simulink model "Grid_Forming_Converters_Microgrid_Github"  (R2020b)
settings: Solver=VariableStepAuto  StartTime=0.0  StopTime=1  RelTol=1e-3
values from neighbouring files (symbols this model uses):
  C_fi_1DG = 50*10^-6    (= 5e-05)    [Script_Primary_Secondary_Controller_GITHUB.m]
  C_fi_2DG = 50*10^-6    (= 5e-05)    [Script_Primary_Secondary_Controller_GITHUB.m]
  C_fi_3DG = 50*10^-6    (= 5e-05)    [Script_Primary_Secondary_Controller_GITHUB.m]
  C_fi_4DG = 50*10^-6    (= 5e-05)    [Script_Primary_Secondary_Controller_GITHUB.m]
  Kff_i_1DG = 0.75    [Script_Primary_Secondary_Controller_GITHUB.m]
  Kff_i_2DG = 0.75    [Script_Primary_Secondary_Controller_GITHUB.m]
  Kff_i_3DG = 0.75    [Script_Primary_Secondary_Controller_GITHUB.m]
  Kff_i_4DG = 0.75    [Script_Primary_Secondary_Controller_GITHUB.m]
  ki = 142500    [Script_Primary_Secondary_Controller_GITHUB.m]
  Kii_1DG = 20000    [Script_Primary_Secondary_Controller_GITHUB.m]
  Kii_2DG = 20000    [Script_Primary_Secondary_Controller_GITHUB.m]
  Kii_3DG = 16000    [Script_Primary_Secondary_Controller_GITHUB.m]
  Kii_4DG = 16000    [Script_Primary_Secondary_Controller_GITHUB.m]
  Kiv_1DG = 420    [Script_Primary_Secondary_Controller_GITHUB.m]
  Kiv_2DG = 420    [Script_Primary_Secondary_Controller_GITHUB.m]
  Kiv_3DG = 390    [Script_Primary_Secondary_Controller_GITHUB.m]
  Kiv_4DG = 390    [Script_Primary_Secondary_Controller_GITHUB.m]
  kp = 285    [Script_Primary_Secondary_Controller_GITHUB.m]
  Kpi_1DG = 15    [Script_Primary_Secondary_Controller_GITHUB.m]
  Kpi_2DG = 15    [Script_Primary_Secondary_Controller_GITHUB.m]
  Kpi_3DG = 10.5    [Script_Primary_Secondary_Controller_GITHUB.m]
  Kpi_4DG = 10.5    [Script_Primary_Secondary_Controller_GITHUB.m]
  Kpv_1DG = 0.1    [Script_Primary_Secondary_Controller_GITHUB.m]
  Kpv_2DG = 0.1    [Script_Primary_Secondary_Controller_GITHUB.m]
  Kpv_3DG = 0.05    [Script_Primary_Secondary_Controller_GITHUB.m]
  Kpv_4DG = 0.05    [Script_Primary_Secondary_Controller_GITHUB.m]
  L_ci_1DG = 0.35*10^-3    (= 0.00035)    [Script_Primary_Secondary_Controller_GITHUB.m]
  L_ci_2DG = 0.35*10^-3    (= 0.00035)    [Script_Primary_Secondary_Controller_GITHUB.m]
  L_fi_1DG = 1.35*10^-3    (= 0.00135)    [Script_Primary_Secondary_Controller_GITHUB.m]
  L_fi_2DG = 1.35*10^-3    (= 0.00135)    [Script_Primary_Secondary_Controller_GITHUB.m]
  L_fi_3DG = 1.35*10^-3    (= 0.00135)    [Script_Primary_Secondary_Controller_GITHUB.m]
  L_fi_4DG = 1.35*10^-3    (= 0.00135)    [Script_Primary_Secondary_Controller_GITHUB.m]
  L_line_1 = 318*10^-6    (= 0.000318)    [Script_Primary_Secondary_Controller_GITHUB.m]
  L_line_2 = 1847*10^-6    (= 0.001847)    [Script_Primary_Secondary_Controller_GITHUB.m]
  L_line_3 = 318*10^-6    (= 0.000318)    [Script_Primary_Secondary_Controller_GITHUB.m]
  L_load_1 = (X_load_1)/(2*pi*f)    (= 0.0477464829276)    [Script_Primary_Secondary_Controller_GITHUB.m]
  L_load_2 = (X_load_2)/(2*pi*f)    (= 0.0318309886184)    [Script_Primary_Secondary_Controller_GITHUB.m]
  L_load_3 = (X_load_3)/(2*pi*f)    (= 0.0318309886184)    [Script_Primary_Secondary_Controller_GITHUB.m]
  L_load_4 = (X_load_4)/(2*pi*f)    (= 0.0477464829276)    [Script_Primary_Secondary_Controller_GITHUB.m]
  m_P_1DG = 9.4*10^-5    (= 9.4e-05)    [Script_Primary_Secondary_Controller_GITHUB.m]
  m_P_2DG = 9.4*10^-5    (= 9.4e-05)    [Script_Primary_Secondary_Controller_GITHUB.m]
  m_P_3DG = 12.5*10^-5    (= 0.000125)    [Script_Primary_Secondary_Controller_GITHUB.m]
  m_P_4DG = 12.5*10^-5    (= 0.000125)    [Script_Primary_Secondary_Controller_GITHUB.m]
  n_Q_1DG = 1.3*10^-3    (= 0.0013)    [Script_Primary_Secondary_Controller_GITHUB.m]
  n_Q_2DG = 1.3*10^-3    (= 0.0013)    [Script_Primary_Secondary_Controller_GITHUB.m]
  n_Q_3DG = 1.5*10^-3    (= 0.0015)    [Script_Primary_Secondary_Controller_GITHUB.m]
  n_Q_4DG = 1.5*10^-3    (= 0.0015)    [Script_Primary_Secondary_Controller_GITHUB.m]
  R_ci_1DG = 0.03    [Script_Primary_Secondary_Controller_GITHUB.m]
  R_ci_2DG = 0.03    [Script_Primary_Secondary_Controller_GITHUB.m]
  R_fi_1DG = 0.1    [Script_Primary_Secondary_Controller_GITHUB.m]
  R_fi_2DG = 0.1    [Script_Primary_Secondary_Controller_GITHUB.m]
  R_fi_3DG = 0.1    [Script_Primary_Secondary_Controller_GITHUB.m]
  R_line_1 = 0.23    [Script_Primary_Secondary_Controller_GITHUB.m]
  R_line_2 = 0.35    [Script_Primary_Secondary_Controller_GITHUB.m]
  R_line_3 = 0.23    [Script_Primary_Secondary_Controller_GITHUB.m]
  R_load_1 = 30    [Script_Primary_Secondary_Controller_GITHUB.m]
  R_load_2 = 20    [Script_Primary_Secondary_Controller_GITHUB.m]
  R_load_3 = 25    [Script_Primary_Secondary_Controller_GITHUB.m]
  R_load_4 = 25    [Script_Primary_Secondary_Controller_GITHUB.m]
  Ts_1DG = 2e-6    (= 2e-06)    [Script_Primary_Secondary_Controller_GITHUB.m]
  w_base_1DG = 2*pi*f_1DG    (= 314.159265359)    [Script_Primary_Secondary_Controller_GITHUB.m]
  w_base_2DG = 2*pi*f_2DG    (= 314.159265359)    [Script_Primary_Secondary_Controller_GITHUB.m]
  w_base_3DG = 2*pi*f_3DG    (= 314.159265359)    [Script_Primary_Secondary_Controller_GITHUB.m]
  w_base_4DG = 2*pi*f_4DG    (= 314.159265359)    [Script_Primary_Secondary_Controller_GITHUB.m]
  wci_1DG = 31.41    [Script_Primary_Secondary_Controller_GITHUB.m]
  wci_2DG = 31.41    [Script_Primary_Secondary_Controller_GITHUB.m]
  wci_3DG = 31.41    [Script_Primary_Secondary_Controller_GITHUB.m]
  wci_4DG = 31.41    [Script_Primary_Secondary_Controller_GITHUB.m]
undefined symbols (not defined in the file or in its folder): L_i_1DG
libraries: powerlib x140, powerlib_meascontrol x68, pid_lib x20
(part 1 of 6)
settings Model: Creator=RI  LastModifiedBy=RI
settings DataIOCC: SaveOutput=off  SaveTime=off  ReturnWorkspaceOutputs=off

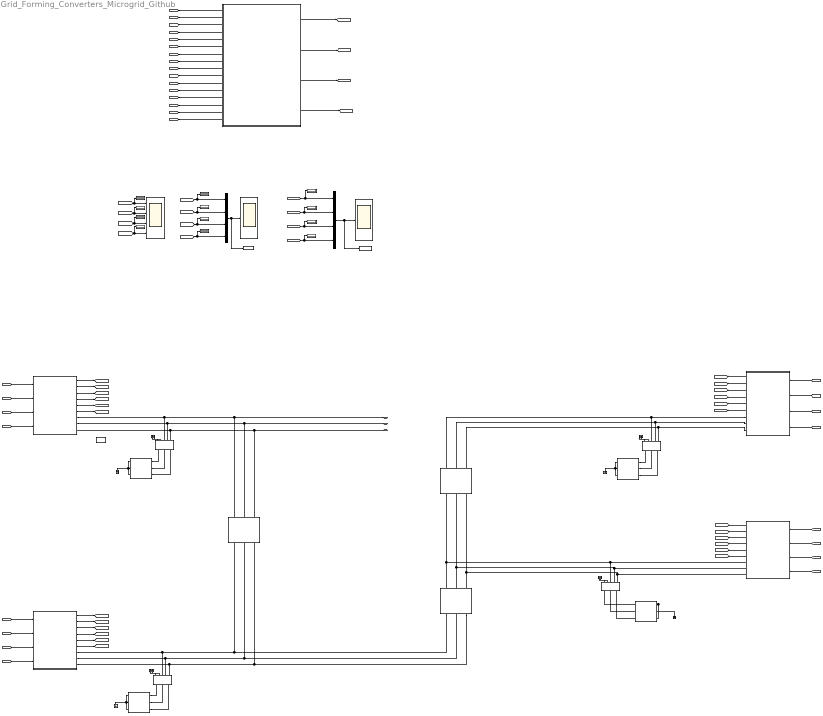
== system Grid_Forming_Converters_Microgrid_Github ==
  " Vo_mag VCVSI" : Scope
  Central Operation Values for VCVSI : Subsystem
  DG 1 VCVSI : Subsystem
  DG 2 VCVSI : Subsystem
  "DG 3 VCVSI " : Subsystem
  "DG 4 VCVSI " : Subsystem
  Display{1..5,12..13,16..19,21} (12 alike) : Display
  Frequency VCVSI : Scope
  Ground{,1..3} (4 alike) : powerlib/Elements/Ground  LConnTagsString=a
  LOAD 1 : powerlib/Elements/Three-Phase Series RLC Branch  LConnTagsString=A|B|C  RConnTagsString=A|B|C  BranchType=RL  Resistance=R_load_1  Inductance=L_load_1  Capacitance=1e-6  Measurements=None
  LOAD 2 : powerlib/Elements/Three-Phase Series RLC Branch  LConnTagsString=A|B|C  RConnTagsString=A|B|C  BranchType=RL  Resistance=R_load_2  Inductance=L_load_2  Capacitance=1e-6  Measurements=None
  LOAD 3 : powerlib/Elements/Three-Phase Series RLC Branch  LConnTagsString=A|B|C  RConnTagsString=A|B|C  BranchType=RL  Resistance=R_load_3  Inductance=L_load_3  Capacitance=1e-6  Measurements=None
  LOAD 4 : powerlib/Elements/Three-Phase Series RLC Branch  LConnTagsString=A|B|C  RConnTagsString=A|B|C  BranchType=RL  Resistance=R_load_4  Inductance=L_load_4  Capacitance=1e-6  Measurements=None
  Mux : Mux
  Mux1 : Mux
  R L Line 1 : powerlib/Elements/Three-Phase Series RLC Branch  LConnTagsString=A|B|C  RConnTagsString=A|B|C  BranchType=RL  Resistance=R_line_1  Inductance=L_line_1  Capacitance=1e-6  Measurements=None
  R L Line 2 : powerlib/Elements/Three-Phase Series RLC Branch  LConnTagsString=A|B|C  RConnTagsString=A|B|C  BranchType=RL  Resistance=R_line_2  Inductance=L_line_2  Capacitance=1e-6  Measurements=None
  R L Line 3 : powerlib/Elements/Three-Phase Series RLC Branch  LConnTagsString=A|B|C  RConnTagsString=A|B|C  BranchType=RL  Resistance=R_line_3  Inductance=L_line_3  Capacitance=1e-6  Measurements=None
  Three-Phase V-I Measurement {1..3,9} (4 alike) : powerlib/Measurements/Three-Phase V-I Measurement  VoltageMeasurement=phase-to-phase  SetLabelV=off  LabelV=Vabc  Vpu=off  VpuLL=off  CurrentMeasurement=yes  SetLabelI=off  LabelI=Iabc  Ipu=off  Pbase=100e6  Vbase=500e3  OutputType=Complex  PhasorSimulation=off  PSBequivalent=0
  To Workspace : ToWorkspace  VariableName=voltages_no_attack  SaveFormat=Timeseries  SampleTime=2e-6
  To Workspace1 : ToWorkspace  VariableName=frequencies_no_attack  SaveFormat=Timeseries  SampleTime=2e-6
  V,I LOAD {1..4} (4 alike) : Scope  NumInputPorts=2
  powergui : powerlib/powergui  Priority=1  SimulationMode=Discrete  SampleTime=2e-6  frequency=60  Iterations=50  frequencyindice=0  Pbase=100e6  ErrMax=1e-4  UnitsV=kV  UnitsW=MW  buscounter=0  FunctionMessages=off  echomessages=off  EnableUseOfTLC=off  CurrentSourceSwitches=off  DisableSnubberDevices=off  DisableRonSwitches=off  DisableVfSwitches=off  DisplayEquations=off  AutomaticDiscreteSolvers=off  SolverType=Tustin/Backward Euler (TBE)  Interpol=off  ExternalGateDelay=off  methode=off  Ts=100  x0status=blocks  SPID=on  SwTol=0  HookPort=off  NonlinearTolerance=1e-4  nMaxIteration=100  ContinueOnMaxIteration=off  RestoreLinks=warning  ResistiveCurrentMeasurement=off  Frange=[0:2:500]  Ylog=off  Xlog=on  ShowGrid=off  save=off  variable=ZData  structure=0  ZoomFFT=off  StartTime=0.0  cycles=1  DisplayStyle=1  fundamental=60  FreqAxis=off  MaxFrequency=1000  frequencyindicesteady=1  RmsSteady=1  display=off
  vod_voltages_VCVSI : Scope  NumInputPorts=4
  A : PMIOPort  Side=Right
  B : PMIOPort  Port=2  Side=Right
  C : PMIOPort  Port=3  Side=Right
  wires:
  DG 1 VCVSI/1(vo_mag_1DG) -> [vo_mag_1DG]
  DG 1 VCVSI/2(v_od_1DG) -> [v_od_1DG]
  DG 1 VCVSI/3(P_1DG) -> [P_1DG]
  DG 1 VCVSI/4(Q_1DG) -> [Q_1DG]
  DG 1 VCVSI/5(w_1DG) -> [w_1DG]
  DG 1 VCVSI/6(frequency_1DG) -> [frequency_1DG]
  [v_od_3DG] -> Display18/1, vod_voltages_VCVSI/3
  [v_od_4DG] -> Display19/1, vod_voltages_VCVSI/4
  [v_od_2DG] -> Display17/1, vod_voltages_VCVSI/2
  [P_2DG] -> Central Operation Values for VCVSI/6(P_2DG)
  Central Operation Values for VCVSI/2(P_matrix) -> [P_matrix]
  [frequency_2DG] -> Mux1/2, Display4/1
  [v_od_2DG] -> Central Operation Values for VCVSI/2(v_od_2DG)
  [vo_mag_2DG] -> Display1/1, Mux/2
  Mux/1 -> To Workspace/1, " Vo_mag VCVSI"/1
  Mux1/1 -> To Workspace1/1, Frequency VCVSI/1
  [vo_mag_4DG] -> Display12/1, Mux/4
  [frequency_1DG] -> Mux1/1, Display3/1
  [frequency_3DG] -> Display5/1, Mux1/3
  [frequency_4DG] -> Display13/1, Mux1/4
  [Q_4DG] -> Central Operation Values for VCVSI/12(Q_4DG)
  [v_od_1DG] -> Display16/1, vod_voltages_VCVSI/1
  [v_od_4DG] -> Central Operation Values for VCVSI/4(v_od_4DG)
  [w_1DG] -> Central Operation Values for VCVSI/13(w_1DG)
  [Q_3DG] -> Central Operation Values for VCVSI/11(Q_3DG)
  [P_3DG] -> Central Operation Values for VCVSI/7(P_3DG)
  [w_3DG] -> Central Operation Values for VCVSI/15(w_3DG)
  [vo_mag_3DG] -> Display2/1, Mux/3
  [w_4DG] -> Central Operation Values for VCVSI/16(w_4DG)
  [Q_1DG] -> Central Operation Values for VCVSI/9(Q_1DG)
  Central Operation Values for VCVSI/3(Q_matrix) -> [Q_matrix]
  Central Operation Values for VCVSI/4(w_matrix) -> [w_matrix]
  [v_od_3DG] -> Central Operation Values for VCVSI/3(v_od_3DG)
  [P_1DG] -> Central Operation Values for VCVSI/5(P_1DG)
  [v_od_1DG] -> Central Operation Values for VCVSI/1(v_od_1DG)
  [Q_2DG] -> Central Operation Values for VCVSI/10(Q_2DG)
  Central Operation Values for VCVSI/1(v_od_matrix) -> [v_od_matrix]
  [P_4DG] -> Central Operation Values for VCVSI/8(P_4DG)
  [vo_mag_1DG] -> Display21/1, Mux/1
  [w_2DG] -> Central Operation Values for VCVSI/14(w_2DG)
  [w_matrix] -> DG 1 VCVSI/4(w_matrix)
  [Q_matrix] -> DG 1 VCVSI/3(Q_matrix)
  [P_matrix] -> DG 1 VCVSI/2(P_matrix)
  [v_od_matrix] -> DG 1 VCVSI/1(v_od_matrix)
  DG 2 VCVSI/5(w_2DG) -> [w_2DG]
  DG 2 VCVSI/2(v_od_2DG) -> [v_od_2DG]
  DG 2 VCVSI/4(Q_2DG) -> [Q_2DG]
  DG 2 VCVSI/3(P_2DG) -> [P_2DG]
  DG 2 VCVSI/1(vo_mag_2DG) -> [vo_mag_2DG]
  DG 2 VCVSI/6(frequency_2DG) -> [frequency_2DG]
  [Q_matrix] -> DG 2 VCVSI/3(Q_matrix)
  [P_matrix] -> DG 2 VCVSI/2(P_matrix)
  [w_matrix] -> DG 2 VCVSI/4(w_matrix)
  [v_od_matrix] -> DG 2 VCVSI/1(v_od_matrix)
  "DG 3 VCVSI "/1(vo_mag_3DG) -> [vo_mag_3DG]
  [Q_matrix] -> "DG 3 VCVSI "/3(Q_matrix)
  "DG 3 VCVSI "/4(Q_3DG) -> [Q_3DG]
  "DG 3 VCVSI "/2(v_od_3DG) -> [v_od_3DG]
  [P_matrix] -> "DG 3 VCVSI "/2(P_matrix)
  "DG 3 VCVSI "/6(frequency_3DG) -> [frequency_3DG]
  "DG 3 VCVSI "/3(P_3DG) -> [P_3DG]
  [w_matrix] -> "DG 3 VCVSI "/4(w_matrix)
  "DG 3 VCVSI "/5(w_3DG) -> [w_3DG]
  [v_od_matrix] -> "DG 3 VCVSI "/1(v_od_matrix)
  [w_matrix] -> "DG 4 VCVSI "/4(w_matrix)
  "DG 4 VCVSI "/6(frequency_4DG) -> [frequency_4DG]
  [P_matrix] -> "DG 4 VCVSI "/2(P_matrix)
  "DG 4 VCVSI "/4(Q_4DG) -> [Q_4DG]
  "DG 4 VCVSI "/2(v_od_4DG) -> [v_od_4DG]
  [v_od_matrix] -> "DG 4 VCVSI "/1(v_od_matrix)
  [Q_matrix] -> "DG 4 VCVSI "/3(Q_matrix)
  "DG 4 VCVSI "/5(w_4DG) -> [w_4DG]
  "DG 4 VCVSI "/3(P_4DG) -> [P_4DG]
  "DG 4 VCVSI "/1(vo_mag_4DG) -> [vo_mag_4DG]
  Three-Phase V-I Measurement 9/1 -> V,I LOAD 1/1
  Three-Phase V-I Measurement 9/2 -> V,I LOAD 1/2
  Three-Phase V-I Measurement 2/1 -> V,I LOAD 2/1
  Three-Phase V-I Measurement 2/2 -> V,I LOAD 2/2
  Three-Phase V-I Measurement 3/2 -> V,I LOAD 4/2
  Three-Phase V-I Measurement 3/1 -> V,I LOAD 4/1
  Three-Phase V-I Measurement 1/2 -> V,I LOAD 3/2
  Three-Phase V-I Measurement 1/1 -> V,I LOAD 3/1
  connections:
  LOAD 1/RConn1 -- Ground/LConn1 -- LOAD 1/RConn3 -- LOAD 1/RConn2
  Three-Phase V-I Measurement 9/RConn1 -- DG 1 VCVSI/RConn1 -- R L Line 1/LConn1 -- A/RConn1
  R L Line 1/LConn2 -- B/RConn1 -- DG 1 VCVSI/RConn2 -- Three-Phase V-I Measurement 9/RConn2
  R L Line 1/LConn3 -- C/RConn1 -- Three-Phase V-I Measurement 9/RConn3 -- DG 1 VCVSI/RConn3
  LOAD 1/LConn3 -- Three-Phase V-I Measurement 9/LConn3
  LOAD 1/LConn1 -- Three-Phase V-I Measurement 9/LConn1
  LOAD 1/LConn2 -- Three-Phase V-I Measurement 9/LConn2
  Three-Phase V-I Measurement 2/RConn1 -- DG 2 VCVSI/RConn1 -- R L Line 2/RConn1 -- R L Line 1/RConn1
  Three-Phase V-I Measurement 2/RConn2 -- DG 2 VCVSI/RConn2 -- R L Line 1/RConn2 -- R L Line 2/RConn2
  LOAD 2/RConn1 -- Ground1/LConn1 -- LOAD 2/RConn3 -- LOAD 2/RConn2
  R L Line 2/RConn3 -- R L Line 1/RConn3 -- DG 2 VCVSI/RConn3 -- Three-Phase V-I Measurement 2/RConn3
  LOAD 2/LConn3 -- Three-Phase V-I Measurement 2/LConn3
  LOAD 2/LConn1 -- Three-Phase V-I Measurement 2/LConn1
  LOAD 2/LConn2 -- Three-Phase V-I Measurement 2/LConn2
  R L Line 3/LConn2 -- Three-Phase V-I Measurement 3/RConn2 -- "DG 4 VCVSI "/RConn2
  Three-Phase V-I Measurement 3/RConn3 -- R L Line 3/LConn3 -- "DG 4 VCVSI "/RConn3
  LOAD 4/RConn1 -- Ground2/LConn1 -- LOAD 4/RConn3 -- LOAD 4/RConn2
  Three-Phase V-I Measurement 3/RConn1 -- R L Line 3/LConn1 -- "DG 4 VCVSI "/RConn1
  LOAD 4/LConn1 -- Three-Phase V-I Measurement 3/LConn1
  LOAD 4/LConn2 -- Three-Phase V-I Measurement 3/LConn2
  LOAD 4/LConn3 -- Three-Phase V-I Measurement 3/LConn3
  Three-Phase V-I Measurement 1/RConn3 -- R L Line 3/RConn3 -- R L Line 2/LConn3 -- "DG 3 VCVSI "/RConn3
  Three-Phase V-I Measurement 1/RConn2 -- R L Line 3/RConn2 -- R L Line 2/LConn2 -- "DG 3 VCVSI "/RConn2
  Three-Phase V-I Measurement 1/RConn1 -- "DG 3 VCVSI "/RConn1 -- R L Line 3/RConn1 -- R L Line 2/LConn1
  LOAD 3/RConn1 -- Ground3/LConn1 -- LOAD 3/RConn2 -- LOAD 3/RConn3
  LOAD 3/LConn1 -- Three-Phase V-I Measurement 1/LConn1
  LOAD 3/LConn3 -- Three-Phase V-I Measurement 1/LConn3
  LOAD 3/LConn2 -- Three-Phase V-I Measurement 1/LConn2

== system Grid_Forming_Converters_Microgrid_Github/Central Operation Values for VCVSI ==
  v_od_1DG : Inport
  v_od_2DG : Inport  Port=2
  v_od_3DG : Inport  Port=3
  v_od_4DG : Inport  Port=4
  P_1DG : Inport  Port=5
  P_2DG : Inport  Port=6
  P_3DG : Inport  Port=7
  P_4DG : Inport  Port=8
  Q_1DG : Inport  Port=9
  Q_2DG : Inport  Port=10
  Q_3DG : Inport  Port=11
  Q_4DG : Inport  Port=12
  w_1DG : Inport  Port=13
  w_2DG : Inport  Port=14
  w_3DG : Inport  Port=15
  w_4DG : Inport  Port=16
  Mux{,1,3..4} (4 alike) : Mux
  v_od_matrix : Outport
  P_matrix : Outport  Port=2
  Q_matrix : Outport  Port=3
  w_matrix : Outport  Port=4
  wires:
  P_1DG/1 -> Mux/1
  P_2DG/1 -> Mux/2
  P_3DG/1 -> Mux/3
  Mux/1 -> P_matrix/1
  Q_2DG/1 -> Mux1/2
  Q_1DG/1 -> Mux1/1
  Q_3DG/1 -> Mux1/3
  Mux1/1 -> Q_matrix/1
  v_od_1DG/1 -> Mux3/1
  v_od_2DG/1 -> Mux3/2
  v_od_3DG/1 -> Mux3/3
  w_2DG/1 -> Mux4/2
  w_1DG/1 -> Mux4/1
  w_3DG/1 -> Mux4/3
  Mux4/1 -> w_matrix/1
  Mux3/1 -> v_od_matrix/1
  P_4DG/1 -> Mux/4
  Q_4DG/1 -> Mux1/4
  w_4DG/1 -> Mux4/4
  v_od_4DG/1 -> Mux3/4

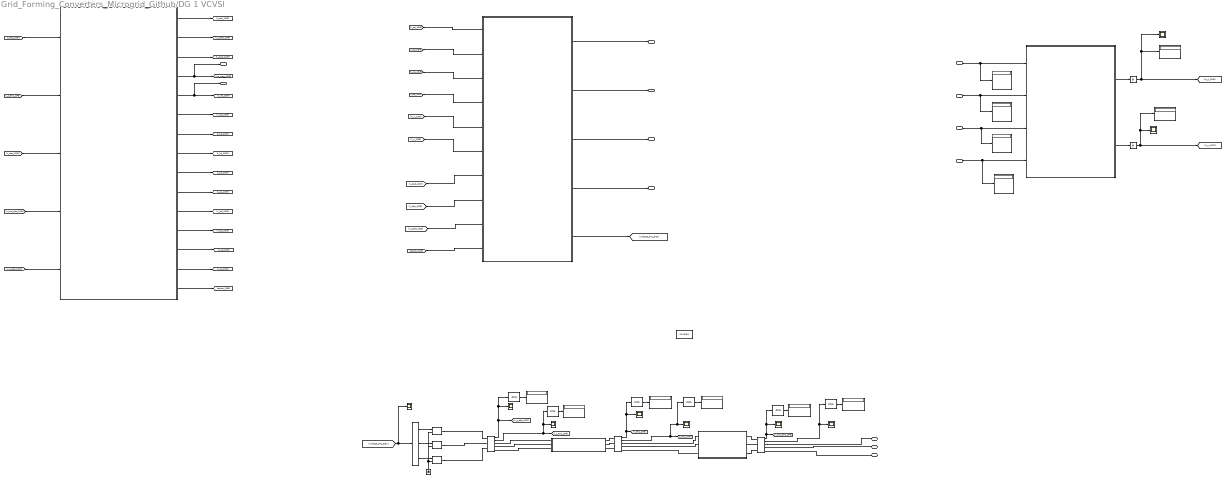
== system Grid_Forming_Converters_Microgrid_Github/DG 1 VCVSI ==
  v_od_matrix : Inport
  P_matrix : Inport  Port=2
  Q_matrix : Inport  Port=3
  w_matrix : Inport  Port=4
  Controlled Voltage Source : powerlib/Electrical Sources/Controlled Voltage Source  Initialize=on  Source_Type=AC  Amplitude=0  Phase=0  Frequency=0  Measurements=None
  Controlled Voltage Source1 : powerlib/Electrical Sources/Controlled Voltage Source  Initialize=on  Source_Type=AC  Amplitude=0  Phase=0  Frequency=0  Measurements=None
  Controlled Voltage Source2 : powerlib/Electrical Sources/Controlled Voltage Source  Initialize=on  Source_Type=AC  Amplitude=0  Phase=0  Frequency=0  Measurements=None
  Conversion and Measurement Block from abc to dq0 frame : Subsystem
  Demux : Demux  Outputs=3
  Display{,1..5,8,11,18..19,22..23} (12 alike) : Display
  Ground : powerlib/Elements/Ground  LConnTagsString=a
  Integrator : Integrator
  Integrator1 : Integrator
  LC FILTER 1 DG : Subsystem
  Primary Controller DG 1 : Subsystem
  RL OUTPUT CONNECTOR 1 DG : Subsystem
  RMS{1..3,5..6} (5 alike) : powerlib_meascontrol/Measurements/RMS  TrueRMS=off  Freq=50  RMSInit=1  Ts=Ts_1DG
  RMS4 : powerlib_meascontrol/Measurements/RMS  TrueRMS=on  Freq=50  RMSInit=1  Ts=Ts_1DG
  Scope : Scope
  Scope3 : Scope
  Secondary Controller DG 1 : MATLAB Function  TreatAsAtomicUnit=on
  Three-Phase V-I Measurement 1 : powerlib/Measurements/Three-Phase V-I Measurement  VoltageMeasurement=phase-to-phase  SetLabelV=off  LabelV=Vabc  Vpu=off  VpuLL=off  CurrentMeasurement=yes  SetLabelI=off  LabelI=Iabc  Ipu=off  Pbase=45000  Vbase=380  OutputType=Complex  PhasorSimulation=off  PSBequivalent=0
  Three-Phase V-I Measurement 2 : powerlib/Measurements/Three-Phase V-I Measurement  VoltageMeasurement=phase-to-phase  SetLabelV=off  LabelV=Vabc  Vpu=off  VpuLL=off  CurrentMeasurement=yes  SetLabelI=off  LabelI=Iabc  Ipu=off  Pbase=45000  Vbase=380  OutputType=Complex  PhasorSimulation=off  PSBequivalent=0
  Three-Phase V-I Measurement 3 : powerlib/Measurements/Three-Phase V-I Measurement  VoltageMeasurement=phase-to-phase  SetLabelV=off  LabelV=Vabc  Vpu=off  VpuLL=off  CurrentMeasurement=yes  SetLabelI=off  LabelI=Iabc  Ipu=off  Pbase=45000  Vbase=380  OutputType=Complex  PhasorSimulation=off  PSBequivalent=0
  i_abc_1DG : Scope
  i_bus_abc_1DG : Scope
  i_s_abc_1DG : Scope
  powergui : powerlib/powergui  Priority=1  SimulationMode=Discrete  SampleTime=2e-6  frequency=60  Iterations=50  frequencyindice=0  Pbase=100e6  ErrMax=1e-4  UnitsV=kV  UnitsW=MW  buscounter=0  FunctionMessages=off  echomessages=off  EnableUseOfTLC=off  CurrentSourceSwitches=off  DisableSnubberDevices=off  DisableRonSwitches=off  DisableVfSwitches=off  DisplayEquations=off  AutomaticDiscreteSolvers=off  SolverType=Tustin/Backward Euler (TBE)  Interpol=off  ExternalGateDelay=off  methode=off  Ts=100  x0status=blocks  SPID=on  SwTol=0  HookPort=off  NonlinearTolerance=1e-4  nMaxIteration=100  ContinueOnMaxIteration=off  RestoreLinks=warning  ResistiveCurrentMeasurement=off  Frange=[0:2:500]  Ylog=off  Xlog=on  ShowGrid=off  save=off  variable=ZData  structure=0  ZoomFFT=off  StartTime=0.0  cycles=1  DisplayStyle=1  fundamental=60  FreqAxis=off  MaxFrequency=1000  frequencyindicesteady=1  RmsSteady=1  display=off
  v_abc_1DG : Scope
  v_bus_abc_1DG : Scope
  v_s_abc_1DG : Scope
  v_s_abc_DG1 : Scope
  A : PMIOPort  Side=Right
  B : PMIOPort  Port=2  Side=Right
  C : PMIOPort  Port=3  Side=Right
  vo_mag_1DG : Outport
  v_od_1DG : Outport  Port=2
  P_1DG : Outport  Port=3
  Q_1DG : Outport  Port=4
  w_1DG : Outport  Port=5
  frequency_1DG : Outport  Port=6
  wires:
  Three-Phase V-I Measurement 2/1 -> RMS1/1, v_abc_1DG/1, [v_abc_1DG]
  Three-Phase V-I Measurement 1/1 -> [v_s_abc_1DG], RMS2/1, v_s_abc_1DG/1
  Three-Phase V-I Measurement 1/2 -> RMS4/1, i_s_abc_1DG/1, [i_s_abc_1DG]
  RMS3/1 -> Display2/1
  Three-Phase V-I Measurement 3/1 -> [v_bus_abc_1DG], v_bus_abc_1DG/1, RMS3/1
  RMS5/1 -> Display4/1
  Three-Phase V-I Measurement 2/2 -> RMS5/1, i_abc_1DG/1, [i_abc_1DG]
  RMS1/1 -> Display/1
  Three-Phase V-I Measurement 3/2 -> RMS6/1, i_bus_abc_1DG/1
  RMS6/1 -> Display5/1
  RMS2/1 -> Display1/1
  RMS4/1 -> Display3/1
  Primary Controller DG 1/1(P_1DG) -> P_1DG/1
  Primary Controller DG 1/5(voltage_abc_DG1) -> [voltage_abc_DG1]
  [V_n_1DG] -> Primary Controller DG 1/6(V_n_1DG)
  Primary Controller DG 1/4(frequency_1DG) -> frequency_1DG/1
  Secondary Controller DG 1/1(v_f_1DG) -> Integrator/1
  Secondary Controller DG 1/2(v_v_1DG) -> Integrator1/1
  Integrator/1 -> [w_n_1DG], Scope/1, Display8/1
  [w_n_1DG] -> Primary Controller DG 1/5(w_n_1DG)
  Integrator1/1 -> Display11/1, Scope3/1, [V_n_1DG]
  [voltage_abc_DG1] -> Demux/1, v_s_abc_DG1/1
  Demux/1 -> Controlled Voltage Source/1
  Demux/2 -> Controlled Voltage Source1/1
  Demux/3 -> Controlled Voltage Source2/1
  [i_abc_1DG] -> Conversion and Measurement Block from abc to dq0 frame/1(i_abc_1DG)
  [i_s_abc_1DG] -> Conversion and Measurement Block from abc to dq0 frame/2(i_s_abc_1DG)
  [v_abc_1DG] -> Conversion and Measurement Block from abc to dq0 frame/3(v_abc_1DG)
  Conversion and Measurement Block from abc to dq0 frame/8(i_1q_1DG) -> [i_1q_1DG]
  Conversion and Measurement Block from abc to dq0 frame/7(i_1d_1DG) -> [i_1d_1DG]
  Conversion and Measurement Block from abc to dq0 frame/6(v_oq_1DG) -> [v_oq_1DG]
  Conversion and Measurement Block from abc to dq0 frame/4(vo_mag_1DG) -> vo_mag_1DG/1, [vo_mag_1DG]
  Conversion and Measurement Block from abc to dq0 frame/5(v_od_1DG) -> v_od_1DG/1, [v_od_1DG]
  [i_oq_1DG] -> Primary Controller DG 1/4(i_oq_1DG)
  [v_od_1DG] -> Primary Controller DG 1/1(v_od_1DG)
  [v_oq_1DG] -> Primary Controller DG 1/3(v_oq_1DG)
  [i_od_1DG] -> Primary Controller DG 1/2(i_od_1DG)
  [i_dq0_1DG] -> Primary Controller DG 1/8(i_dq0_1DG)
  [v_dq0_1DG] -> Primary Controller DG 1/7(v_dq0_1DG)
  [i_s_dq0_1DG] -> Primary Controller DG 1/9(i_s_dq0_1DG)
  Conversion and Measurement Block from abc to dq0 frame/9(i_od_1DG) -> [i_od_1DG]
  Conversion and Measurement Block from abc to dq0 frame/10(i_oq_1DG) -> [i_oq_1DG]
  Conversion and Measurement Block from abc to dq0 frame/15(alpha_1DG) -> [alpha_1DG]
  Conversion and Measurement Block from abc to dq0 frame/1(i_dq0_1DG) -> [i_dq0_1DG]
  Conversion and Measurement Block from abc to dq0 frame/2(i_s_dq0_1DG) -> [i_s_dq0_1DG]
  Conversion and Measurement Block from abc to dq0 frame/3(v_dq0_1DG) -> [v_dq0_1DG]
  [alpha_1DG] -> Primary Controller DG 1/10(alpha_1DG)
  Primary Controller DG 1/3(w_1DG) -> w_1DG/1
  Primary Controller DG 1/2(Q_1DG) -> Q_1DG/1
  w_matrix/1 -> Display23/1, Secondary Controller DG 1/4(w_matrix)
  Q_matrix/1 -> Display22/1, Secondary Controller DG 1/3(Q_matrix)
  P_matrix/1 -> Display19/1, Secondary Controller DG 1/2(P_matrix)
  v_od_matrix/1 -> Display18/1, Secondary Controller DG 1/1(v_od_matrix)
  [v_bus_abc_1DG] -> Conversion and Measurement Block from abc to dq0 frame/4(v_bus_abc_1DG)
  Conversion and Measurement Block from abc to dq0 frame/12(v_bq_1DG) -> [v_bq_1DG]
  Conversion and Measurement Block from abc to dq0 frame/11(v_bd_1DG) -> [v_bd_1DG]
  [v_s_abc_1DG] -> Conversion and Measurement Block from abc to dq0 frame/5(v_s_abc_1DG)
  Conversion and Measurement Block from abc to dq0 frame/13(v_id_1DG) -> [v_id_1DG]
  Conversion and Measurement Block from abc to dq0 frame/14(v_iq_1DG) -> [v_iq_1DG]
  connections:
  RL OUTPUT CONNECTOR 1 DG/LConn2 -- Three-Phase V-I Measurement 2/RConn2
  LC FILTER 1 DG/LConn2 -- Three-Phase V-I Measurement 1/RConn2
  RL OUTPUT CONNECTOR 1 DG/LConn1 -- Three-Phase V-I Measurement 2/RConn1
  C/RConn1 -- Three-Phase V-I Measurement 3/RConn3
  Three-Phase V-I Measurement 2/LConn3 -- LC FILTER 1 DG/RConn3
  Three-Phase V-I Measurement 3/RConn1 -- A/RConn1
  B/RConn1 -- Three-Phase V-I Measurement 3/RConn2
  Controlled Voltage Source1/RConn1 -- Three-Phase V-I Measurement 1/LConn2
  RL OUTPUT CONNECTOR 1 DG/LConn3 -- Three-Phase V-I Measurement 2/RConn3
  Three-Phase V-I Measurement 3/LConn1 -- RL OUTPUT CONNECTOR 1 DG/RConn1
  Three-Phase V-I Measurement 2/LConn1 -- LC FILTER 1 DG/RConn1
  Three-Phase V-I Measurement 3/LConn2 -- RL OUTPUT CONNECTOR 1 DG/RConn2
  RL OUTPUT CONNECTOR 1 DG/RConn3 -- Three-Phase V-I Measurement 3/LConn3
  Controlled Voltage Source2/RConn1 -- Three-Phase V-I Measurement 1/LConn3
  LC FILTER 1 DG/LConn3 -- Three-Phase V-I Measurement 1/RConn3
  LC FILTER 1 DG/LConn1 -- Three-Phase V-I Measurement 1/RConn1
  Three-Phase V-I Measurement 2/LConn2 -- LC FILTER 1 DG/RConn2
  Controlled Voltage Source/RConn1 -- Three-Phase V-I Measurement 1/LConn1
  Ground/LConn1 -- Controlled Voltage Source/LConn1 -- Controlled Voltage Source1/LConn1 -- Controlled Voltage Source2/LConn1

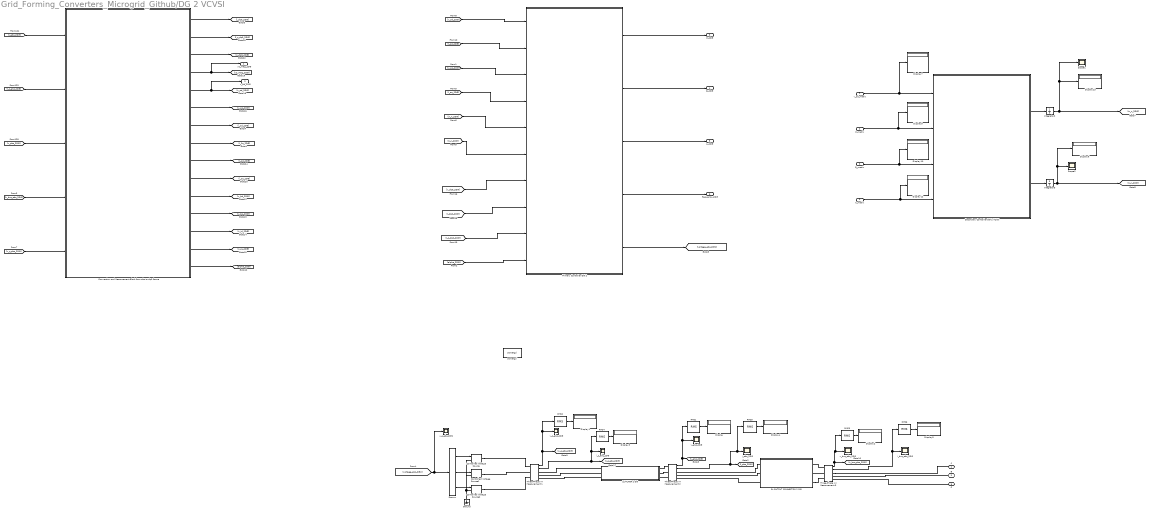
== system Grid_Forming_Converters_Microgrid_Github/DG 2 VCVSI ==
  v_od_matrix : Inport
  P_matrix : Inport  Port=2
  Q_matrix : Inport  Port=3
  w_matrix : Inport  Port=4
  Controlled Voltage Source : powerlib/Electrical Sources/Controlled Voltage Source  Initialize=on  Source_Type=AC  Amplitude=0  Phase=0  Frequency=0  Measurements=None
  Controlled Voltage Source1 : powerlib/Electrical Sources/Controlled Voltage Source  Initialize=on  Source_Type=AC  Amplitude=0  Phase=0  Frequency=0  Measurements=None
  Controlled Voltage Source2 : powerlib/Electrical Sources/Controlled Voltage Source  Initialize=on  Source_Type=AC  Amplitude=0  Phase=0  Frequency=0  Measurements=None
  Conversion and Measurement Block from abc to dq0 frame : Subsystem
  Demux : Demux  Outputs=3
  Display{,1..7,9..10,12..13} (12 alike) : Display
  Ground : powerlib/Elements/Ground  LConnTagsString=a
  Integrator2 : Integrator
  Integrator3 : Integrator
  LC FILTER 2 DG : Subsystem
  Primary Controller DG 2 : Subsystem
  RL OUTPUT CONNECTOR 2 DG : Subsystem
  RMS{1..3,5..6} (5 alike) : powerlib_meascontrol/Measurements/RMS  TrueRMS=off  Freq=50  RMSInit=1  Ts=Ts_1DG
  RMS4 : powerlib_meascontrol/Measurements/RMS  TrueRMS=on  Freq=50  RMSInit=1  Ts=Ts_1DG
  Scope1 : Scope
  Scope2 : Scope
  Secondary Controller DG 2 VCVSI : MATLAB Function  TreatAsAtomicUnit=on
  Three-Phase V-I Measurement 1 : powerlib/Measurements/Three-Phase V-I Measurement  VoltageMeasurement=phase-to-phase  SetLabelV=off  LabelV=Vabc  Vpu=off  VpuLL=off  CurrentMeasurement=yes  SetLabelI=off  LabelI=Iabc  Ipu=off  Pbase=45000  Vbase=380  OutputType=Complex  PhasorSimulation=off  PSBequivalent=0
  Three-Phase V-I Measurement 2 : powerlib/Measurements/Three-Phase V-I Measurement  VoltageMeasurement=phase-to-phase  SetLabelV=off  LabelV=Vabc  Vpu=off  VpuLL=off  CurrentMeasurement=yes  SetLabelI=off  LabelI=Iabc  Ipu=off  Pbase=45000  Vbase=380  OutputType=Complex  PhasorSimulation=off  PSBequivalent=0
  Three-Phase V-I Measurement 3 : powerlib/Measurements/Three-Phase V-I Measurement  VoltageMeasurement=phase-to-phase  SetLabelV=off  LabelV=Vabc  Vpu=off  VpuLL=off  CurrentMeasurement=yes  SetLabelI=off  LabelI=Iabc  Ipu=off  Pbase=45000  Vbase=380  OutputType=Complex  PhasorSimulation=off  PSBequivalent=0
  i_abc_2DG : Scope
  i_bus_abc_2DG : Scope
  i_s_abc_2DG : Scope
  powergui : powerlib/powergui  Priority=1  SimulationMode=Discrete  SampleTime=2e-6  frequency=60  Iterations=50  frequencyindice=0  Pbase=100e6  ErrMax=1e-4  UnitsV=kV  UnitsW=MW  buscounter=0  FunctionMessages=off  echomessages=off  EnableUseOfTLC=off  CurrentSourceSwitches=off  DisableSnubberDevices=off  DisableRonSwitches=off  DisableVfSwitches=off  DisplayEquations=off  AutomaticDiscreteSolvers=off  SolverType=Tustin/Backward Euler (TBE)  Interpol=off  ExternalGateDelay=off  methode=off  Ts=100  x0status=blocks  SPID=on  SwTol=0  HookPort=off  NonlinearTolerance=1e-4  nMaxIteration=100  ContinueOnMaxIteration=off  RestoreLinks=warning  ResistiveCurrentMeasurement=off  Frange=[0:2:500]  Ylog=off  Xlog=on  ShowGrid=off  save=off  variable=ZData  structure=0  ZoomFFT=off  StartTime=0.0  cycles=1  DisplayStyle=1  fundamental=60  FreqAxis=off  MaxFrequency=1000  frequencyindicesteady=1  RmsSteady=1  display=off
  v_abc_2DG : Scope
  v_bus_abc_2DG : Scope
  v_s_abc_2DG : Scope
  v_s_abc_DG2 : Scope
  A : PMIOPort  Side=Right
  B : PMIOPort  Port=2  Side=Right
  C : PMIOPort  Port=3  Side=Right
  vo_mag_2DG : Outport
  v_od_2DG : Outport  Port=2
  P_2DG : Outport  Port=3
  Q_2DG : Outport  Port=4
  w_2DG : Outport  Port=5
  frequency_2DG : Outport  Port=6
  wires:
  Three-Phase V-I Measurement 2/1 -> RMS1/1, v_abc_2DG/1, [v_abc_2DG]
  Three-Phase V-I Measurement 1/1 -> [v_s_abc_2DG], RMS2/1, v_s_abc_2DG/1
  Three-Phase V-I Measurement 1/2 -> RMS4/1, i_s_abc_2DG/1, [i_s_abc_2DG]
  RMS3/1 -> Display2/1
  Three-Phase V-I Measurement 3/1 -> [v_bus_abc_2DG], RMS3/1, v_bus_abc_2DG/1
  RMS5/1 -> Display4/1
  Three-Phase V-I Measurement 2/2 -> RMS5/1, i_abc_2DG/1, [i_abc_2DG]
  RMS1/1 -> Display/1
  Three-Phase V-I Measurement 3/2 -> RMS6/1, i_bus_abc_2DG/1
  RMS6/1 -> Display5/1
  RMS2/1 -> Display1/1
  RMS4/1 -> Display3/1
  Primary Controller DG 2/1(P_2DG) -> P_2DG/1
  Primary Controller DG 2/5(voltage_abc_DG2) -> [voltage_abc_DG2]
  [V_n_2DG] -> Primary Controller DG 2/6(V_n_2DG)
  Primary Controller DG 2/4(frequency_2DG) -> frequency_2DG/1
  [w_n_2DG] -> Primary Controller DG 2/5(w_n_2DG)
  [voltage_abc_DG2] -> Demux/1, v_s_abc_DG2/1
  Demux/1 -> Controlled Voltage Source/1
  Demux/2 -> Controlled Voltage Source1/1
  Demux/3 -> Controlled Voltage Source2/1
  [i_abc_2DG] -> Conversion and Measurement Block from abc to dq0 frame/1(i_abc_2DG)
  [i_s_abc_2DG] -> Conversion and Measurement Block from abc to dq0 frame/2(i_s_abc_2DG)
  [v_abc_2DG] -> Conversion and Measurement Block from abc to dq0 frame/3(v_abc_2DG)
  Conversion and Measurement Block from abc to dq0 frame/8(i_1q_2DG) -> [i_1q_2DG]
  Conversion and Measurement Block from abc to dq0 frame/7(i_1d_2DG) -> [i_1d_2DG]
  Conversion and Measurement Block from abc to dq0 frame/6(v_oq_2DG) -> [v_oq_2DG]
  Conversion and Measurement Block from abc to dq0 frame/4(vo_mag_2DG) -> [vo_mag_2DG], vo_mag_2DG/1
  Conversion and Measurement Block from abc to dq0 frame/5(v_od_2DG) -> [v_od_2DG], v_od_2DG/1
  [i_oq_2DG] -> Primary Controller DG 2/4(i_oq_2DG)
  [v_od_2DG] -> Primary Controller DG 2/1(v_od_2DG)
  [v_oq_2DG] -> Primary Controller DG 2/3(v_oq_2DG)
  [i_od_2DG] -> Primary Controller DG 2/2(i_od_2DG)
  [i_dq0_2DG] -> Primary Controller DG 2/8(i_dq0_2DG)
  [v_dq0_2DG] -> Primary Controller DG 2/7(v_dq0_2DG)
  [i_s_dq0_2DG] -> Primary Controller DG 2/9(i_s_dq0_2DG)
  Conversion and Measurement Block from abc to dq0 frame/9(i_od_2DG) -> [i_od_2DG]
  Conversion and Measurement Block from abc to dq0 frame/10(i_oq_2DG) -> [i_oq_2DG]
  Conversion and Measurement Block from abc to dq0 frame/15(alpha_2DG) -> [alpha_2DG]
  Conversion and Measurement Block from abc to dq0 frame/1(i_dq0_2DG) -> [i_dq0_2DG]
  Conversion and Measurement Block from abc to dq0 frame/2(i_s_dq0_2DG) -> [i_s_dq0_2DG]
  Conversion and Measurement Block from abc to dq0 frame/3(v_dq0_2DG) -> [v_dq0_2DG]
  [alpha_2DG] -> Primary Controller DG 2/10(alpha_2DG)
  Primary Controller DG 2/3(w_2DG) -> w_2DG/1
  Primary Controller DG 2/2(Q_2DG) -> Q_2DG/1
  Secondary Controller DG 2 VCVSI/2(v_v_2DG) -> Integrator3/1
  w_matrix/1 -> Secondary Controller DG 2 VCVSI/4(w_matrix), Display12/1
  Integrator2/1 -> [w_n_2DG], Scope1/1, Display13/1
  Secondary Controller DG 2 VCVSI/1(v_f_2DG) -> Integrator2/1
  Integrator3/1 -> [V_n_2DG], Display6/1, Scope2/1
  v_od_matrix/1 -> Secondary Controller DG 2 VCVSI/1(v_od_matrix), Display7/1
  Q_matrix/1 -> Secondary Controller DG 2 VCVSI/3(Q_matrix), Display10/1
  P_matrix/1 -> Secondary Controller DG 2 VCVSI/2(P_matrix), Display9/1
  [v_bus_abc_2DG] -> Conversion and Measurement Block from abc to dq0 frame/4(v_bus_abc_2DG)
  [v_s_abc_2DG] -> Conversion and Measurement Block from abc to dq0 frame/5(v_s_abc_2DG)
  Conversion and Measurement Block from abc to dq0 frame/11(v_bd_2DG) -> [v_bd_2DG]
  Conversion and Measurement Block from abc to dq0 frame/12(v_bq_2DG) -> [v_bq_2DG]
  Conversion and Measurement Block from abc to dq0 frame/14(v_iq_2DG) -> [v_iq_2DG]
  Conversion and Measurement Block from abc to dq0 frame/13(v_id_2DG) -> [v_id_2DG]
  connections:
  RL OUTPUT CONNECTOR 2 DG/LConn2 -- Three-Phase V-I Measurement 2/RConn2
  LC FILTER 2 DG/LConn2 -- Three-Phase V-I Measurement 1/RConn2
  RL OUTPUT CONNECTOR 2 DG/LConn1 -- Three-Phase V-I Measurement 2/RConn1
  C/RConn1 -- Three-Phase V-I Measurement 3/RConn3
  Three-Phase V-I Measurement 2/LConn3 -- LC FILTER 2 DG/RConn3
  Three-Phase V-I Measurement 3/RConn1 -- A/RConn1
  B/RConn1 -- Three-Phase V-I Measurement 3/RConn2
  Controlled Voltage Source1/RConn1 -- Three-Phase V-I Measurement 1/LConn2
  RL OUTPUT CONNECTOR 2 DG/LConn3 -- Three-Phase V-I Measurement 2/RConn3
  Three-Phase V-I Measurement 3/LConn1 -- RL OUTPUT CONNECTOR 2 DG/RConn1
  Three-Phase V-I Measurement 2/LConn1 -- LC FILTER 2 DG/RConn1
  Three-Phase V-I Measurement 3/LConn2 -- RL OUTPUT CONNECTOR 2 DG/RConn2
  RL OUTPUT CONNECTOR 2 DG/RConn3 -- Three-Phase V-I Measurement 3/LConn3
  Controlled Voltage Source2/RConn1 -- Three-Phase V-I Measurement 1/LConn3
  LC FILTER 2 DG/LConn3 -- Three-Phase V-I Measurement 1/RConn3
  LC FILTER 2 DG/LConn1 -- Three-Phase V-I Measurement 1/RConn1
  Three-Phase V-I Measurement 2/LConn2 -- LC FILTER 2 DG/RConn2
  Controlled Voltage Source/RConn1 -- Three-Phase V-I Measurement 1/LConn1
  Ground/LConn1 -- Controlled Voltage Source/LConn1 -- Controlled Voltage Source1/LConn1 -- Controlled Voltage Source2/LConn1

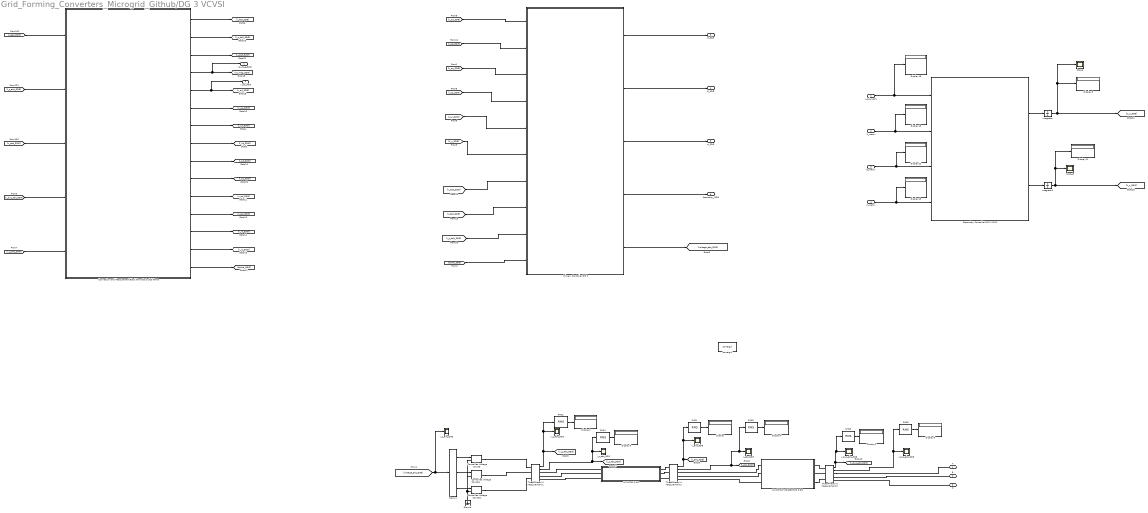
== system Grid_Forming_Converters_Microgrid_Github/DG 3 VCVSI  ==
  v_od_matrix : Inport
  P_matrix : Inport  Port=2
  Q_matrix : Inport  Port=3
  w_matrix : Inport  Port=4
  Controlled Voltage Source : powerlib/Electrical Sources/Controlled Voltage Source  Initialize=on  Source_Type=AC  Amplitude=0  Phase=0  Frequency=0  Measurements=None
  Controlled Voltage Source1 : powerlib/Electrical Sources/Controlled Voltage Source  Initialize=on  Source_Type=AC  Amplitude=0  Phase=0  Frequency=0  Measurements=None
  Controlled Voltage Source2 : powerlib/Electrical Sources/Controlled Voltage Source  Initialize=on  Source_Type=AC  Amplitude=0  Phase=0  Frequency=0  Measurements=None
  Conversion and Measurement Block from abc to dq0 frame : Subsystem
  Demux : Demux  Outputs=3
  Display{,1..5,8,11,18..19,22..23} (12 alike) : Display
  Ground : powerlib/Elements/Ground  LConnTagsString=a
  Integrator : Integrator
  Integrator1 : Integrator
  LC FILTER 3 DG : Subsystem
  Primary Controller DG 3 : Subsystem
  RL OUTPUT CONNECTOR 3 DG : Subsystem
  RMS{1..3,5..6} (5 alike) : powerlib_meascontrol/Measurements/RMS  TrueRMS=off  Freq=50  RMSInit=1  Ts=Ts_1DG
  RMS4 : powerlib_meascontrol/Measurements/RMS  TrueRMS=on  Freq=50  RMSInit=1  Ts=Ts_1DG
  Scope : Scope
  Scope3 : Scope
  Secondary Controller DG 3 VCVSI : MATLAB Function  TreatAsAtomicUnit=on
  Three-Phase V-I Measurement 1 : powerlib/Measurements/Three-Phase V-I Measurement  VoltageMeasurement=phase-to-phase  SetLabelV=off  LabelV=Vabc  Vpu=off  VpuLL=off  CurrentMeasurement=yes  SetLabelI=off  LabelI=Iabc  Ipu=off  Pbase=45000  Vbase=380  OutputType=Complex  PhasorSimulation=off  PSBequivalent=0
  Three-Phase V-I Measurement 2 : powerlib/Measurements/Three-Phase V-I Measurement  VoltageMeasurement=phase-to-phase  SetLabelV=off  LabelV=Vabc  Vpu=off  VpuLL=off  CurrentMeasurement=yes  SetLabelI=off  LabelI=Iabc  Ipu=off  Pbase=45000  Vbase=380  OutputType=Complex  PhasorSimulation=off  PSBequivalent=0
  Three-Phase V-I Measurement 3 : powerlib/Measurements/Three-Phase V-I Measurement  VoltageMeasurement=phase-to-phase  SetLabelV=off  LabelV=Vabc  Vpu=off  VpuLL=off  CurrentMeasurement=yes  SetLabelI=off  LabelI=Iabc  Ipu=off  Pbase=45000  Vbase=380  OutputType=Complex  PhasorSimulation=off  PSBequivalent=0
  i_abc_3DG : Scope
  i_bus_abc_3DG : Scope
  i_s_abc_3DG : Scope
  powergui : powerlib/powergui  Priority=1  SimulationMode=Discrete  SampleTime=2e-6  frequency=60  Iterations=50  frequencyindice=0  Pbase=100e6  ErrMax=1e-4  UnitsV=kV  UnitsW=MW  buscounter=0  FunctionMessages=off  echomessages=off  EnableUseOfTLC=off  CurrentSourceSwitches=off  DisableSnubberDevices=off  DisableRonSwitches=off  DisableVfSwitches=off  DisplayEquations=off  AutomaticDiscreteSolvers=off  SolverType=Tustin/Backward Euler (TBE)  Interpol=off  ExternalGateDelay=off  methode=off  Ts=100  x0status=blocks  SPID=on  SwTol=0  HookPort=off  NonlinearTolerance=1e-4  nMaxIteration=100  ContinueOnMaxIteration=off  RestoreLinks=warning  ResistiveCurrentMeasurement=off  Frange=[0:2:500]  Ylog=off  Xlog=on  ShowGrid=off  save=off  variable=ZData  structure=0  ZoomFFT=off  StartTime=0.0  cycles=1  DisplayStyle=1  fundamental=60  FreqAxis=off  MaxFrequency=1000  frequencyindicesteady=1  RmsSteady=1  display=off
  v_abc_3DG : Scope
  v_bus_abc_3DG : Scope
  v_s_abc_3DG : Scope
  v_s_abc_DG3 : Scope
  A : PMIOPort  Side=Right
  B : PMIOPort  Port=2  Side=Right
  C : PMIOPort  Port=3  Side=Right
  vo_mag_3DG : Outport
  v_od_3DG : Outport  Port=2
  P_3DG : Outport  Port=3
  Q_3DG : Outport  Port=4
  w_3DG : Outport  Port=5
  frequency_3DG : Outport  Port=6
  wires:
  Three-Phase V-I Measurement 2/1 -> RMS1/1, v_abc_3DG/1, [v_abc_3DG]
  Three-Phase V-I Measurement 1/1 -> [v_s_abc_3DG], RMS2/1, v_s_abc_3DG/1
  Three-Phase V-I Measurement 1/2 -> RMS4/1, i_s_abc_3DG/1, [i_s_abc_3DG]
  RMS3/1 -> Display2/1
  Three-Phase V-I Measurement 3/1 -> [v_bus_abc_3DG], RMS3/1, v_bus_abc_3DG/1
  RMS5/1 -> Display4/1
  Three-Phase V-I Measurement 2/2 -> RMS5/1, i_abc_3DG/1, [i_abc_3DG]
  RMS1/1 -> Display/1
  Three-Phase V-I Measurement 3/2 -> RMS6/1, i_bus_abc_3DG/1
  RMS6/1 -> Display5/1
  RMS2/1 -> Display1/1
  RMS4/1 -> Display3/1
  Primary Controller DG 3/1(P_3DG) -> P_3DG/1
  Primary Controller DG 3/5(voltage_abc_DG3) -> [voltage_abc_DG3]
  [V_n_3DG] -> Primary Controller DG 3/6(V_n_3DG)
  Primary Controller DG 3/4(frequency_3DG) -> frequency_3DG/1
  [w_n_3DG] -> Primary Controller DG 3/5(w_n_3DG)
  [voltage_abc_DG3] -> Demux/1, v_s_abc_DG3/1
  Demux/1 -> Controlled Voltage Source/1
  Demux/2 -> Controlled Voltage Source1/1
  Demux/3 -> Controlled Voltage Source2/1
  [i_abc_3DG] -> Conversion and Measurement Block from abc to dq0 frame/1(i_abc_3DG)
  [i_s_abc_3DG] -> Conversion and Measurement Block from abc to dq0 frame/2(i_s_abc_3DG)
  [v_abc_3DG] -> Conversion and Measurement Block from abc to dq0 frame/3(v_abc_3DG)
  Conversion and Measurement Block from abc to dq0 frame/8(i_1q_3DG) -> [i_1q_3DG]
  Conversion and Measurement Block from abc to dq0 frame/7(i_1d_3DG) -> [i_1d_3DG]
  Conversion and Measurement Block from abc to dq0 frame/6(v_oq_3DG) -> [v_oq_3DG]
  Conversion and Measurement Block from abc to dq0 frame/4(vo_mag_3DG) -> [vo_mag_3DG], vo_mag_3DG/1
  Conversion and Measurement Block from abc to dq0 frame/5(v_od_3DG) -> [v_od_3DG], v_od_3DG/1
  [i_oq_3DG] -> Primary Controller DG 3/4(i_oq_3DG)
  [v_od_3DG] -> Primary Controller DG 3/1(v_od_3DG)
  [v_oq_3DG] -> Primary Controller DG 3/3(v_oq_3DG)
  [i_od_3DG] -> Primary Controller DG 3/2(i_od_3DG)
  [i_dq0_3DG] -> Primary Controller DG 3/8(i_dq0_3DG)
  [v_dq0_3DG] -> Primary Controller DG 3/7(v_dq0_3DG)
  [i_s_dq0_3DG] -> Primary Controller DG 3/9(i_s_dq0_3DG)
  Conversion and Measurement Block from abc to dq0 frame/9(i_od_3DG) -> [i_od_3DG]
  Conversion and Measurement Block from abc to dq0 frame/10(i_oq_3DG) -> [i_oq_3DG]
  Conversion and Measurement Block from abc to dq0 frame/15(alpha_3DG) -> [alpha_3DG]
  Conversion and Measurement Block from abc to dq0 frame/1(i_dq0_3DG) -> [i_dq0_3DG]
  Conversion and Measurement Block from abc to dq0 frame/2(i_s_dq0_3DG) -> [i_s_dq0_3DG]
  Conversion and Measurement Block from abc to dq0 frame/3(v_dq0_3DG) -> [v_dq0_3DG]
  [alpha_3DG] -> Primary Controller DG 3/10(alpha_3DG)
  Primary Controller DG 3/3(w_3DG) -> w_3DG/1
  Primary Controller DG 3/2(Q_3DG) -> Q_3DG/1
  [v_bus_abc_3DG] -> Conversion and Measurement Block from abc to dq0 frame/4(v_bus_abc_3DG)
  [v_s_abc_3DG] -> Conversion and Measurement Block from abc to dq0 frame/5(v_s_abc_3DG)
  Conversion and Measurement Block from abc to dq0 frame/11(v_bd_3DG) -> [v_bd_3DG]
  Conversion and Measurement Block from abc to dq0 frame/12(v_bq_3DG) -> [v_bq_3DG]
  Conversion and Measurement Block from abc to dq0 frame/14(v_iq_3DG) -> [v_iq_3DG]
  Conversion and Measurement Block from abc to dq0 frame/13(v_id_3DG) -> [v_id_3DG]
  Secondary Controller DG 3 VCVSI/1(v_f_3DG) -> Integrator/1
  Secondary Controller DG 3 VCVSI/2(v_v_3DG) -> Integrator1/1
  Integrator1/1 -> Display11/1, Scope3/1, [V_n_3DG]
  Integrator/1 -> [w_n_3DG], Scope/1, Display8/1
  v_od_matrix/1 -> Display18/1, Secondary Controller DG 3 VCVSI/1(v_od_matrix)
  P_matrix/1 -> Display19/1, Secondary Controller DG 3 VCVSI/2(P_matrix)
  Q_matrix/1 -> Display22/1, Secondary Controller DG 3 VCVSI/3(Q_matrix)
  w_matrix/1 -> Display23/1, Secondary Controller DG 3 VCVSI/4(w_matrix)
  connections:
  RL OUTPUT CONNECTOR 3 DG/LConn2 -- Three-Phase V-I Measurement 2/RConn2
  LC FILTER 3 DG/LConn2 -- Three-Phase V-I Measurement 1/RConn2
  RL OUTPUT CONNECTOR 3 DG/LConn1 -- Three-Phase V-I Measurement 2/RConn1
  C/RConn1 -- Three-Phase V-I Measurement 3/RConn3
  Three-Phase V-I Measurement 2/LConn3 -- LC FILTER 3 DG/RConn3
  Three-Phase V-I Measurement 3/RConn1 -- A/RConn1
  B/RConn1 -- Three-Phase V-I Measurement 3/RConn2
  Controlled Voltage Source1/RConn1 -- Three-Phase V-I Measurement 1/LConn2
  RL OUTPUT CONNECTOR 3 DG/LConn3 -- Three-Phase V-I Measurement 2/RConn3
  Three-Phase V-I Measurement 3/LConn1 -- RL OUTPUT CONNECTOR 3 DG/RConn1
  Three-Phase V-I Measurement 2/LConn1 -- LC FILTER 3 DG/RConn1
  Three-Phase V-I Measurement 3/LConn2 -- RL OUTPUT CONNECTOR 3 DG/RConn2
  RL OUTPUT CONNECTOR 3 DG/RConn3 -- Three-Phase V-I Measurement 3/LConn3
  Controlled Voltage Source2/RConn1 -- Three-Phase V-I Measurement 1/LConn3
  LC FILTER 3 DG/LConn3 -- Three-Phase V-I Measurement 1/RConn3
  LC FILTER 3 DG/LConn1 -- Three-Phase V-I Measurement 1/RConn1
  Three-Phase V-I Measurement 2/LConn2 -- LC FILTER 3 DG/RConn2
  Controlled Voltage Source/RConn1 -- Three-Phase V-I Measurement 1/LConn1
  Ground/LConn1 -- Controlled Voltage Source/LConn1 -- Controlled Voltage Source1/LConn1 -- Controlled Voltage Source2/LConn1
